simulink model "TeamA_PAsqualo"  (R2020a)
settings: Solver=VariableStepAuto  StartTime=0.0  StopTime=stop_time  FixedStep=0.05  RelTol=1e-3
InitFcn:
  | main_init
values from neighbouring files (symbols this model uses):
  a1 = rho * D^4 * alpha1    (= 0.000388302366464)    [main_init.m]
  a2 = -rho * D^3 * alpha2 * (1 - omega)    (= 0.0037030698432)    [main_init.m]
  ag = [Ax Ay Az]'    [init_modello.m]
  alpha1 = 0.0113    [main_init.m]
  alpha2 = -0.0091    [main_init.m]
  areaOfInterestCorner = [42.317744;10.915136; 0]    [init_controllo.m]    (also in missionA.m = [42.317744)
  bg = [Bx By Bz]'    [init_modello.m]
  cd_pitch = 0.7    [init_modello.m]
  cd_roll = 0.04    [init_modello.m]
  cd_x = 0.4    [init_modello.m]
  cd_y = 1    [init_modello.m]
  cd_yaw = 0.7    [init_modello.m]
  cd_z = 1    [init_modello.m]
  cg = [Cx Cy Cz]'    [init_modello.m]
  D = 0.076    [main_init.m]
  dead_zone_limit = 31.5    [main_init.m]
  dg = [Dx Dy Dz]'    [init_modello.m]
  eg = [Ex Ey Ez]'    [init_modello.m]
  fg = [Fx Fy Fz]'    [init_modello.m]
  g = 9.81    [init_modello.m]
  galleggiamento = 7.6786    [init_controllo.m]
  gg = [Gx Gy Gz]'    [init_modello.m]
  H0 = 0    [init_modello.m]
  init_position = [pointP(1),pointP(2),0.15,0,0,deg2rad(alpha)]'    [init_modello.m]
  init_velocity = [0 0 0 0 0 0]'    [init_modello.m]
  initial_state_cov = blkdiag(diag(cov_gps(1,1:2)), cov_depth*eye(n_state_filter-2))    [init_navigazione.m]
  Ixx = 0.93304097392    [init_modello.m]
  Ixy = 0    [init_modello.m]
  Ixz = 0    [init_modello.m]
  Iyy = 25.58745481378    (= 25.5874548138)    [init_modello.m]
  Iyz = 0    [init_modello.m]
  Izz = 25.58745481378    (= 25.5874548138)    [init_modello.m]
  K_i_heave_div = 20    [init_controllo.m]
  K_i_heave_pos = 1    [init_controllo.m]
  K_i_heave_surf = 20    [init_controllo.m]
  K_i_heave_trans = 5    [init_controllo.m]
  K_i_heave_turn = 5    [init_controllo.m]
  K_i_pitch_div = 0    [init_controllo.m]
  K_i_pitch_pos = 0    [init_controllo.m]
  K_i_pitch_surf = 0    [init_controllo.m]
  K_i_pitch_trans = 0    [init_controllo.m]
  K_i_pitch_turn = 0    [init_controllo.m]
  K_i_roll_div = 0    [init_controllo.m]
  K_i_roll_pos = 0    [init_controllo.m]
  K_i_roll_surf = 1    [init_controllo.m]
  K_i_roll_trans = 0    [init_controllo.m]
  K_i_roll_turn = 0    [init_controllo.m]
  K_i_surge_div = 3    [init_controllo.m]
  K_i_surge_pos = 5    [init_controllo.m]
  K_i_surge_surf = 3    [init_controllo.m]
  K_i_surge_trans = 2.5    [init_controllo.m]
  K_i_surge_turn = 10    [init_controllo.m]
  K_i_sway_div = 6    [init_controllo.m]
  K_i_sway_pos = 5    [init_controllo.m]
  K_i_sway_surf = 3    [init_controllo.m]
  K_i_sway_trans = 6    [init_controllo.m]
  K_i_sway_turn = 50    [init_controllo.m]
  K_i_yaw_div = 0    [init_controllo.m]
  K_i_yaw_pos = 1    [init_controllo.m]
  K_i_yaw_surf = 0    [init_controllo.m]
  K_i_yaw_trans = 20    [init_controllo.m]
  K_p_heave_div = 200    [init_controllo.m]
  K_p_heave_pos = 350    [init_controllo.m]
  K_p_heave_surf = 200    [init_controllo.m]
  K_p_heave_trans = 200    [init_controllo.m]
  K_p_heave_turn = 200    [init_controllo.m]
  K_p_phi_div = 0.15    [init_controllo.m]
  K_p_phi_pos = 0.1    [init_controllo.m]
  K_p_phi_surf = 0.15    [init_controllo.m]
  K_p_phi_trans = 0.1    [init_controllo.m]
  K_p_phi_turn = 0.1    [init_controllo.m]
  K_p_pitch_div = 50    [init_controllo.m]
  K_p_pitch_pos = 25    [init_controllo.m]
  K_p_pitch_surf = 50    [init_controllo.m]
  K_p_pitch_trans = 25    [init_controllo.m]
  K_p_pitch_turn = 25    [init_controllo.m]
  K_p_psi_div = 0.3    [init_controllo.m]
  K_p_psi_pos = 0.25    [init_controllo.m]
  K_p_psi_surf = 0.3    [init_controllo.m]
  K_p_psi_trans = 0.2    [init_controllo.m]
  K_p_roll_div = 10    [init_controllo.m]
  K_p_roll_pos = 4    [init_controllo.m]
  K_p_roll_surf = 10    [init_controllo.m]
  K_p_roll_trans = 4    [init_controllo.m]
  K_p_roll_turn = 4    [init_controllo.m]
  K_p_surge_div = 80    [init_controllo.m]
  K_p_surge_pos = 34.5    [init_controllo.m]
  K_p_surge_surf = 80    [init_controllo.m]
  K_p_surge_trans = 40    [init_controllo.m]
  K_p_surge_turn = 150    [init_controllo.m]
  K_p_sway_div = 100    [init_controllo.m]
  K_p_sway_pos = 90    [init_controllo.m]
  K_p_sway_surf = 80    [init_controllo.m]
  K_p_sway_trans = 90    [init_controllo.m]
  K_p_sway_turn = 200    [init_controllo.m]
  K_p_th_div = 0.3    [init_controllo.m]
  K_p_th_pos = 0.1    [init_controllo.m]
  K_p_th_surf = 0.3    [init_controllo.m]
  K_p_th_trans = 0.1    [init_controllo.m]
  K_p_th_turn = 0.1    [init_controllo.m]
  K_p_x_div = 0.12    [init_controllo.m]
  K_p_x_pos = 0.12    [init_controllo.m]
  K_p_x_surf = 0.12    [init_controllo.m]
  K_p_y_div = 0.6    [init_controllo.m]
  K_p_y_pos = 0.34    [init_controllo.m]
  K_p_y_surf = 0.1    [init_controllo.m]
  K_p_y_trans = 0.3    [init_controllo.m]
  K_p_y_turn = 0.3    [init_controllo.m]
  K_p_yaw_div = 70    [init_controllo.m]
  K_p_yaw_pos = 20    [init_controllo.m]
  K_p_yaw_surf = 70    [init_controllo.m]
  K_p_yaw_trans = 160    [init_controllo.m]
  K_p_z_div = 0.35    [init_controllo.m]
  K_p_z_pos = 0.2    [init_controllo.m]
  K_p_z_surf = 0.35    [init_controllo.m]
  K_p_z_trans = 0.7    [init_controllo.m]
  K_p_z_turn = 0.7    [init_controllo.m]
  Kadd = 0    [init_modello.m]
  m = 106    [init_modello.m]
  Madd = -((((1/5)*(b^2-a^2)^2))*(alpha_0-beta_0))/((((2*(b^2-a^2)^2))+(b^2-a^2)^2)*(alpha_0-beta_0)*m)    [init_modello.m]
  ... (+59 more)
undefined symbols (not defined in the file or in its folder): DiscIntNeverNeededParam, initial_state
libraries: simulink x2, vrlib x1
(part 5 of 5)

== matlab function TeamA_PAsqualo/controller/positioning controller/sway_controller/Sway PID controller/compute_position_errors ==
  data: enable input; err_pos output; ref input; est_state input; areaOfInterestCorner parameter
function err_pos = fcn(enable, ref, est_state,areaOfInterestCorner)
references_NED = zeros(3,1);
est_state_NED  = zeros(3,1);
phi = est_state(4);
th  = est_state(5);
psi = est_state(6);
coder.extrinsic('evalin','wgs84Ellipsoid','geodetic2ned');   
orig = [areaOfInterestCorner(1)   areaOfInterestCorner(2)   areaOfInterestCorner(3)]'; %origine terna NED
wgs84 = wgs84Ellipsoid;
if enable == 1
    % Cambiamento di riferimento da WGS84 a NED frame
   [x_ref, y_ref, z_ref] = geodetic2ned(ref(1),ref(2),ref(3),orig(1),orig(2),orig(3),wgs84);
   references_NED = [x_ref, y_ref, z_ref]';
   [x_est, y_est, z_est] = geodetic2ned(est_state(1),est_state(2),est_state(3),orig(1),orig(2),orig(3),wgs84);
   est_state_NED  =  [x_est, y_est, est_state(3)]';
   % Calcolo errore posizione da NED a BODY frame
   err_NED  = references_NED - est_state_NED;
   %
   R_z_psi = [cos(psi)    sin(psi)     0;
              -sin(psi)   cos(psi)     0;
                 0           0         1];
          
   R_y_th =  [cos(th)        0      -sin(th);
                 0           1         0;
              sin(th)        0       cos(th)];
       
   R_x_phi = [   1           0             0;
                 0         cos(phi)    sin(phi);
                 0        -sin(phi)    cos(phi)];
          
   R_NB = ((R_z_psi')*(R_y_th')*(R_x_phi'))'; % matrice rotazione NED->BODY
   err_pos_BODY = R_NB * err_NED;
   err_pos = err_pos_BODY(2);
else 
   err_pos = 0;
end
end

== matlab function TeamA_PAsqualo/controller/positioning controller/sway_controller/Sway PID controller/compute_velocity_error ==
  data: enable input; err_vel output; v_des input; est_meas input
function err_vel = fcn(enable,v_des,est_meas)
if enable == 1
   err_vel =  v_des - est_meas(8);

else 
    err_vel = 0;
end
end

== matlab function TeamA_PAsqualo/controller/positioning controller/yaw_controller/Yaw PID controller/compute_orientation_errors ==
  data: enable input; err_orient output; ref input; est_state input
function err_orient = fcn(enable, ref, est_state)
coder.extrinsic('wrapToPi');
err_orient = 0;
phi = est_state(4);
th  = est_state(5);
%
J_inv = [1       0          -sin(th); 
         0   cos(phi)  cos(th)*sin(phi);
         0  -sin(phi)  cos(th)*cos(phi)];
if enable == 1
   err_orient_1 = wrapToPi(J_inv*([ref(4);ref(5);ref(6)] -...
                           [est_state(4);est_state(5);est_state(6)]));
else 
   err_orient_1 = zeros(3,1);
end
err_orient = err_orient_1(3);
end

== matlab function TeamA_PAsqualo/controller/positioning controller/yaw_controller/Yaw PID controller/compute_velocity_error ==
  data: enable input; err_vel output; v_des input; est_meas input
function err_vel = fcn(enable,v_des,est_meas)
if enable == 1
   err_vel =  v_des - est_meas(12);
else
    err_vel = 0;
end
end

== matlab function TeamA_PAsqualo/controller/surfacing controller/heave_controller/Heave PID controller/compute_position_errors ==
  data: enable input; err_pos output; ref input; est_state input; w_des output; areaOfInterestCorner parameter
function [err_pos, w_des] = fcn(enable, ref, est_state,areaOfInterestCorner)
references_NED = zeros(3,1);
est_state_NED  = zeros(3,1);
phi = est_state(4);
th  = est_state(5);
psi = est_state(6);
coder.extrinsic('evalin','wgs84Ellipsoid','geodetic2ned');
orig = [areaOfInterestCorner(1)   areaOfInterestCorner(2)   areaOfInterestCorner(3)]'; %origine terna NED
wgs84 = wgs84Ellipsoid;
err_pos = 0;
w_des = 0;
if enable == 1
    % Cambiamento di riferimento da WGS84 a NED frame
   [x_ref, y_ref, z_ref] = geodetic2ned(ref(1),ref(2),ref(3),orig(1),orig(2),orig(3),wgs84);
   references_NED = [x_ref, y_ref, z_ref]';
   [x_est, y_est, z_est] = geodetic2ned(est_state(1),est_state(2),est_state(3),orig(1),orig(2),orig(3),wgs84);
   est_state_NED  =  [x_est, y_est, z_est]';
   est_state_NED = [est_state_NED(1);est_state_NED(2);est_state(3)];
   % Calcolo errore posizione da NED a BODY frame
   err_NED  = references_NED - est_state_NED;
   R_z_psi = [cos(psi)    sin(psi)     0;
              -sin(psi)   cos(psi)     0;
                 0           0         1];
          
   R_y_th =  [cos(th)        0      -sin(th);
                 0           1         0;
              sin(th)        0       cos(th)];
       
   R_x_phi = [   1           0             0;
                 0         cos(phi)    sin(phi);
                 0        -sin(phi)    cos(phi)];
          
   R_NB = ((R_z_psi')*(R_y_th')*(R_x_phi'))';
   err_pos_BODY = R_NB * err_NED;
   offset = -0.5;  % metri di distanza dal punto desiderato
   if err_pos_BODY(3) < offset
       err_pos = 0;
       w_des   = ref(9);
   end
   if err_pos_BODY(3) > offset
       err_pos = err_pos_BODY(3);
       w_des   = 0;
   end
else
   err_pos = 0;
   w_des   = 0;
end
end

== matlab function TeamA_PAsqualo/controller/surfacing controller/pitch_controller/Pitch PID controller/compute_orientation_errors ==
  data: enable input; err_orient output; ref input; est_state input
function err_orient = fcn(enable, ref, est_state)
coder.extrinsic('wrapToPi');
err_orient = 0;
phi = est_state(4);
th  = est_state(5);
%
J_inv = [1       0          -sin(th); 
         0   cos(phi)  cos(th)*sin(phi);
         0  -sin(phi)  cos(th)*cos(phi)];
if enable == 1
   err_orient_1 = wrapToPi(J_inv*([ref(4);ref(5);ref(6)] -...
                           [est_state(4);est_state(5);est_state(6)]));
else 
   err_orient_1 = zeros(3,1);
end
err_orient = err_orient_1(2);
end

== matlab function TeamA_PAsqualo/controller/surfacing controller/pitch_controller/Pitch PID controller/compute_velocity_error ==
  data: enable input; err_vel output; v_des input; est_meas input
function err_vel = fcn(enable,v_des,est_meas)
if enable == 1
   err_vel =  v_des - est_meas(11);
else
    err_vel = 0;
end
end

== matlab function TeamA_PAsqualo/controller/surfacing controller/heave_controller/Heave PID controller/compute_velocity_error ==
  data: enable input; err_vel output; v_des input; est_meas input
function err_vel = fcn(enable,v_des,est_meas)
if enable == 1
   err_vel =  v_des - est_meas(9);
else
    err_vel = 0;
end
end

== matlab function TeamA_PAsqualo/controller/surfacing controller/roll_controller/Roll PID controller/compute_orientation_errors ==
  data: enable input; err_orient output; ref input; est_state input
function err_orient = fcn(enable, ref, est_state)
coder.extrinsic('wrapToPi');
err_orient = 0;
phi = est_state(4);
th  = est_state(5);
%
J_inv = [1       0          -sin(th); 
         0   cos(phi)  cos(th)*sin(phi);
         0  -sin(phi)  cos(th)*cos(phi)];
if enable == 1
   err_orient_1 = wrapToPi(J_inv*([ref(4);ref(5);ref(6)] -...
                           [est_state(4);est_state(5);est_state(6)]));
else 
   err_orient_1 = zeros(3,1);
end
err_orient = err_orient_1(1);
end

== matlab function TeamA_PAsqualo/controller/surfacing controller/roll_controller/Roll PID controller/compute_velocity_error ==
  data: enable input; err_vel output; v_des input; est_meas input
function err_vel = fcn(enable,v_des,est_meas)
if enable == 1
   err_vel =  v_des - est_meas(10);
else
    err_vel = 0;
end
end

== matlab function TeamA_PAsqualo/controller/surfacing controller/surge_controller/Surge PID controller/compute_position_errors ==
  data: enable input; err_pos output; ref input; est_state input; areaOfInterestCorner parameter
function err_pos = fcn(enable, ref, est_state,areaOfInterestCorner)
references_NED = zeros(3,1);
est_state_NED  = zeros(3,1);
phi = est_state(4);
th  = est_state(5);
psi = est_state(6);
coder.extrinsic('evalin','wgs84Ellipsoid','geodetic2ned');
orig = [areaOfInterestCorner(1)   areaOfInterestCorner(2)   areaOfInterestCorner(3)]'; %origine terna NED
wgs84 = wgs84Ellipsoid;
if enable == 1
    % Cambiamento di riferimento da WGS84 a NED frame
   [x_ref, y_ref, z_ref] = geodetic2ned(ref(1),ref(2),ref(3),orig(1),orig(2),orig(3),wgs84);
   references_NED = [x_ref, y_ref, z_ref]';
   [x_est, y_est, z_est] = geodetic2ned(est_state(1),est_state(2),est_state(3),orig(1),orig(2),orig(3),wgs84);
   est_state_NED  =  [x_est, y_est, est_state(3)]';
   % Calcolo errore posizione da NED a BODY frame
   err_NED  = references_NED - est_state_NED;
   R_z_psi = [cos(psi)    sin(psi)     0;
              -sin(psi)   cos(psi)     0;
                 0           0         1];
          
   R_y_th =  [cos(th)        0      -sin(th);
                 0           1         0;
              sin(th)        0       cos(th)];
       
   R_x_phi = [   1           0             0;
                 0         cos(phi)    sin(phi);
                 0        -sin(phi)    cos(phi)];
          
   R_NB = ((R_z_psi')*(R_y_th')*(R_x_phi'))';
   err_pos_BODY = R_NB * err_NED;
   err_pos = err_pos_BODY(1);
else
   err_pos = 0;
end
end

== matlab function TeamA_PAsqualo/controller/surfacing controller/surge_controller/Surge PID controller/compute_velocity_error ==
  data: enable input; err_vel output; v_des input; est_meas input
function err_vel = fcn(enable,v_des,est_meas)
if enable == 1
   err_vel =  v_des - est_meas(7);
else
    err_vel = 0;
end
end

== matlab function TeamA_PAsqualo/controller/surfacing controller/sway_controller/Sway PID controller/compute_position_errors ==
  data: enable input; err_pos output; ref input; est_state input; areaOfInterestCorner parameter
function err_pos = fcn(enable, ref, est_state,areaOfInterestCorner)
references_NED = zeros(3,1);
est_state_NED  = zeros(3,1);
phi = est_state(4);
th  = est_state(5);
psi = est_state(6);
coder.extrinsic('evalin','wgs84Ellipsoid','geodetic2ned');
orig = [areaOfInterestCorner(1)   areaOfInterestCorner(2)   areaOfInterestCorner(3)]'; %origine terna NED
wgs84 = wgs84Ellipsoid;
if enable == 1
    % Cambiamento di riferimento da WGS84 a NED frame
   [x_ref, y_ref, z_ref] = geodetic2ned(ref(1),ref(2),ref(3),orig(1),orig(2),orig(3),wgs84);
   references_NED = [x_ref, y_ref, z_ref]';
   [x_est, y_est, z_est] = geodetic2ned(est_state(1),est_state(2),est_state(3),orig(1),orig(2),orig(3),wgs84);
   est_state_NED  =  [x_est, y_est,est_state(3)]';
   % Calcolo errore posizione da NED a BODY frame
   err_NED  = references_NED - est_state_NED;
   R_z_psi = [cos(psi)    sin(psi)     0;
              -sin(psi)   cos(psi)     0;
                 0           0         1];
          
   R_y_th =  [cos(th)        0      -sin(th);
                 0           1         0;
              sin(th)        0       cos(th)];
       
   R_x_phi = [   1           0             0;
                 0         cos(phi)    sin(phi);
                 0        -sin(phi)    cos(phi)];
          
   R_NB = ((R_z_psi')*(R_y_th')*(R_x_phi'))';
   err_pos_BODY = R_NB * err_NED;
   err_pos = err_pos_BODY(2);
else
   err_pos = 0;
end
end

== matlab function TeamA_PAsqualo/controller/surfacing controller/sway_controller/Sway PID controller/compute_velocity_error ==
  data: enable input; err_vel output; v_des input; est_meas input
function err_vel = fcn(enable,v_des,est_meas)
if enable == 1
   err_vel =  v_des - est_meas(8);
else
    err_vel = 0;
end
end

== matlab function TeamA_PAsqualo/controller/surfacing controller/yaw_controller/Yaw PID controller/compute_orientation_errors ==
  data: enable input; err_orient output; ref input; est_state input
function err_orient = fcn(enable, ref, est_state)
coder.extrinsic('wrapToPi');
err_orient = 0;
phi = est_state(4);
th  = est_state(5);
%
J_inv = [1       0          -sin(th); 
         0   cos(phi)  cos(th)*sin(phi);
         0  -sin(phi)  cos(th)*cos(phi)];
if enable == 1
   err_orient_1 = wrapToPi(J_inv*([ref(4);ref(5);ref(6)] -...
                           [est_state(4);est_state(5);est_state(6)]));
else 
   err_orient_1 = zeros(3,1);
end
err_orient = err_orient_1(3);
end

== matlab function TeamA_PAsqualo/controller/surfacing controller/yaw_controller/Yaw PID controller/compute_velocity_error ==
  data: enable input; err_vel output; v_des input; est_meas input
function err_vel = fcn(enable,v_des,est_meas)
if enable == 1
   err_vel =  v_des - est_meas(12);
else
    err_vel = 0;
end
end

== matlab function TeamA_PAsqualo/controller/transect controller/heave_controller/Heave PID controller/compute_position_errors ==
  data: enable input; err_pos output; ref input; est_state input; areaOfInterestCorner parameter
function err_pos = fcn(enable, ref, est_state,areaOfInterestCorner)
references_NED = zeros(3,1);
est_state_NED  = zeros(3,1);
phi = est_state(4);
th  = est_state(5);
psi = est_state(6);
coder.extrinsic('evalin','wgs84Ellipsoid','geodetic2ned');
orig = [areaOfInterestCorner(1)   areaOfInterestCorner(2)   areaOfInterestCorner(3)]'; %origine terna NED
wgs84 = wgs84Ellipsoid;
if enable == 1
    % Cambiamento di riferimento da WGS84 a NED frame
   [x_ref, y_ref, z_ref] = geodetic2ned(ref(1),ref(2),ref(3),orig(1),orig(2),orig(3),wgs84);
   references_NED = [x_ref, y_ref, z_ref]';
   [x_est, y_est, z_est] = geodetic2ned(est_state(1),est_state(2),est_state(3),orig(1),orig(2),orig(3),wgs84);
   est_state_NED  =  [x_est, y_est, z_est]';
   est_state_NED = [est_state_NED(1);est_state_NED(2);est_state(3)];
   % Calcolo errore posizione da NED a BODY frame
   err_NED  = references_NED - est_state_NED;
   R_z_psi = [cos(psi)    sin(psi)     0;
              -sin(psi)   cos(psi)     0;
                 0           0         1];
          
   R_y_th =  [cos(th)        0      -sin(th);
                 0           1         0;
              sin(th)        0       cos(th)];
       
   R_x_phi = [   1           0             0;
                 0         cos(phi)    sin(phi);
                 0        -sin(phi)    cos(phi)];
          
   R_NB = ((R_z_psi')*(R_y_th')*(R_x_phi'))';
   err_pos_BODY = R_NB * err_NED;
   err_pos = err_pos_BODY(3);
else
   err_pos = 0;
end
end

== matlab function TeamA_PAsqualo/controller/transect controller/heave_controller/Heave PID controller/compute_velocity_error ==
  data: enable input; err_vel output; v_des input; est_meas input
function err_vel = fcn(enable,v_des,est_meas)
if enable == 1
   err_vel =  v_des - est_meas(9);
else
    err_vel = 0;
end
end

== matlab function TeamA_PAsqualo/controller/transect controller/pitch_controller/Pitch PID controller/compute_orientation_errors ==
  data: enable input; err_orient output; ref input; est_state input
function err_orient = fcn(enable, ref, est_state)
coder.extrinsic('wrapToPi');
err_orient = 0;
phi = est_state(4);
th  = est_state(5);
%
J_inv = [1       0          -sin(th); 
         0   cos(phi)  cos(th)*sin(phi);
         0  -sin(phi)  cos(th)*cos(phi)];
if enable == 1
   err_orient_1 = wrapToPi(J_inv*([ref(4);ref(5);ref(6)] -...
                           [est_state(4);est_state(5);est_state(6)]));
else 
   err_orient_1 = zeros(3,1);
end
err_orient = err_orient_1(2);
end

== matlab function TeamA_PAsqualo/controller/transect controller/pitch_controller/Pitch PID controller/compute_velocity_error ==
  data: enable input; err_vel output; v_des input; est_meas input
function err_vel = fcn(enable,v_des,est_meas)
if enable == 1
   err_vel =  v_des - est_meas(11);
else
    err_vel = 0;
end
end

== matlab function TeamA_PAsqualo/controller/transect controller/roll_controller/Roll PID controller/compute_orientation_errors ==
  data: enable input; err_orient output; ref input; est_state input
function err_orient = fcn(enable, ref, est_state)
coder.extrinsic('wrapToPi');
err_orient = 0;
phi = est_state(4);
th  = est_state(5);
%
J_inv = [1       0          -sin(th); 
         0   cos(phi)  cos(th)*sin(phi);
         0  -sin(phi)  cos(th)*cos(phi)];
if enable == 1
   err_orient_1 = wrapToPi(J_inv*([ref(4);ref(5);ref(6)] -...
                           [est_state(4);est_state(5);est_state(6)]));
else 
   err_orient_1 = zeros(3,1);
end
err_orient = err_orient_1(1);
end

== matlab function TeamA_PAsqualo/controller/transect controller/roll_controller/Roll PID controller/compute_velocity_error ==
  data: enable input; err_vel output; v_des input; est_meas input
function err_vel = fcn(enable,v_des,est_meas)
if enable == 1
   err_vel =  v_des - est_meas(10);
else
    err_vel = 0;
end
end

== matlab function TeamA_PAsqualo/controller/transect controller/surge_controller/Surge PID controller/ compute_velocity_error ==
  data: enable input; ref input; est_meas input; err_vel output
function err_vel = fcn(enable, ref, est_meas)
if  enable == 1
    err_vel = ref(7) - est_meas(7);
else
    err_vel = 0;
end
end

== matlab function TeamA_PAsqualo/controller/transect controller/sway_controller/Sway PID controller/compute_position_errors ==
  data: enable input; err_pos output; ref input; est_state input; areaOfInterestCorner parameter
function err_pos = fcn(enable, ref, est_state,areaOfInterestCorner)
coder.extrinsic('wrapToPi');
coder.extrinsic('evalin','wgs84Ellipsoid','geodetic2ned');
references_NED = zeros(3,1);
est_state_NED  = zeros(3,1);
phi = est_state(4);
th  = est_state(5);
psi = est_state(6);
psi = wrapToPi(psi);
orig = [areaOfInterestCorner(1)   areaOfInterestCorner(2)   areaOfInterestCorner(3)]'; %origine terna NED
wgs84 = wgs84Ellipsoid;
if enable == 1
    % Cambiamento di riferimento da WGS84 a NED frame
   [x_ref, y_ref, z_ref] = geodetic2ned(ref(1),ref(2),ref(3),orig(1),orig(2),orig(3),wgs84);
   references_NED = [x_ref, y_ref, z_ref]';
   [x_est, y_est, z_est] = geodetic2ned(est_state(1),est_state(2),est_state(3),orig(1),orig(2),orig(3),wgs84);
   est_state_NED  =  [x_est, y_est, est_state(3)]';
   % Calcolo errore posizione da NED a BODY frame
   err_NED  = references_NED - est_state_NED;
   R_z_psi = [cos(psi)    sin(psi)     0;
              -sin(psi)   cos(psi)     0;
                 0           0         1];
          
   R_y_th =  [cos(th)        0      -sin(th);
                 0           1         0;
              sin(th)        0       cos(th)];
       
   R_x_phi = [   1           0             0;
                 0         cos(phi)    sin(phi);
                 0        -sin(phi)    cos(phi)];
          
   R_NB = ((R_z_psi')*(R_y_th')*(R_x_phi'))';
   err_pos_BODY = R_NB * err_NED;
   err_pos = err_pos_BODY(2);
else
   err_pos = 0;
end
end

== matlab function TeamA_PAsqualo/controller/transect controller/sway_controller/Sway PID controller/compute_velocity_error ==
  data: enable input; err_vel output; v_des input; est_meas input
function err_vel = fcn(enable,v_des,est_meas)
if enable == 1
   err_vel =  v_des - est_meas(8);
else
    err_vel = 0;
end
end

== matlab function TeamA_PAsqualo/controller/transect controller/yaw_controller/Yaw PID controller/compute_orientation_errors ==
  data: enable input; err_orient output; ref input; est_state input
function err_orient = fcn(enable, ref, est_state)
coder.extrinsic('wrapToPi');
err_orient = 0;
phi = est_state(4);
th  = est_state(5);
%
J_inv = [1       0          -sin(th); 
         0   cos(phi)  cos(th)*sin(phi);
         0  -sin(phi)  cos(th)*cos(phi)];
if enable == 1
   err_orient_1 = wrapToPi(J_inv*([ref(4);ref(5);ref(6)] -...
                           [est_state(4);est_state(5);est_state(6)]));
else 
   err_orient_1 = zeros(3,1);
end
err_orient = err_orient_1(3);
end

== matlab function TeamA_PAsqualo/controller/transect controller/yaw_controller/Yaw PID controller/compute_velocity_error ==
  data: enable input; err_vel output; v_des input; est_meas input
function err_vel = fcn(enable,v_des,est_meas)
if enable == 1
   err_vel =  v_des - est_meas(12);
else
    err_vel = 0;
end
end

== matlab function TeamA_PAsqualo/controller/turning controller/heave_controller/Heave PID controller/compute_position_errors ==
  data: enable input; err_pos output; ref input; est_state input; areaOfInterestCorner parameter
function err_pos = fcn(enable, ref, est_state,areaOfInterestCorner)
references_NED = zeros(3,1);
est_state_NED  = zeros(3,1);
phi = est_state(4);
th  = est_state(5);
psi = est_state(6);
coder.extrinsic('evalin','wgs84Ellipsoid','geodetic2ned');
orig = [areaOfInterestCorner(1)   areaOfInterestCorner(2)   areaOfInterestCorner(3)]'; %origine terna NED
wgs84 = wgs84Ellipsoid;
if enable == 1
   % Cambiamento di riferimento da WGS84 a NED frame
   [x_ref, y_ref, z_ref] = geodetic2ned(ref(1),ref(2),ref(3),orig(1),orig(2),orig(3),wgs84);
   references_NED = [x_ref, y_ref, z_ref]';
   [x_est, y_est, z_est] = geodetic2ned(est_state(1),est_state(2),est_state(3),orig(1),orig(2),orig(3),wgs84);
   est_state_NED  =  [x_est, y_est, z_est]';
   est_state_NED = [est_state_NED(1);est_state_NED(2);est_state(3)];
   % Calcolo errore posizione da NED a BODY frame
   err_NED  = references_NED - est_state_NED;
   R_z_psi = [cos(psi)    sin(psi)     0;
              -sin(psi)   cos(psi)     0;
                 0           0         1];
          
   R_y_th =  [cos(th)        0      -sin(th);
                 0           1         0;
              sin(th)        0       cos(th)];
       
   R_x_phi = [   1           0             0;
                 0         cos(phi)    sin(phi);
                 0        -sin(phi)    cos(phi)];
          
   R_NB = ((R_z_psi')*(R_y_th')*(R_x_phi'))';
   err_pos_BODY = R_NB * err_NED;
   err_pos = err_pos_BODY(3);
else
   err_pos = 0;
end
end

== matlab function TeamA_PAsqualo/controller/turning controller/heave_controller/Heave PID controller/compute_velocity_error ==
  data: enable input; err_vel output; v_des input; est_meas input
function err_vel = fcn(enable,v_des,est_meas)
if enable == 1
   err_vel =  v_des - est_meas(9);
else
    err_vel = 0;
end
end

== matlab function TeamA_PAsqualo/controller/turning controller/pitch_controller/Pitch PID controller/compute_orientation_errors ==
  data: enable input; err_orient output; ref input; est_state input
function err_orient = fcn(enable, ref, est_state)
coder.extrinsic('wrapToPi');
err_orient = 0;
phi = est_state(4);
th  = est_state(5);
%
J_inv = [1       0          -sin(th); 
         0   cos(phi)  cos(th)*sin(phi);
         0  -sin(phi)  cos(th)*cos(phi)];
if enable == 1
   err_orient_1 = wrapToPi(J_inv*([ref(4);ref(5);ref(6)] -...
                           [est_state(4);est_state(5);est_state(6)]));
else 
   err_orient_1 = zeros(3,1);
end
err_orient = err_orient_1(2);
end

== matlab function TeamA_PAsqualo/controller/turning controller/pitch_controller/Pitch PID controller/compute_velocity_error ==
  data: enable input; err_vel output; v_des input; est_meas input
function err_vel = fcn(enable,v_des,est_meas)
if enable == 1
   err_vel =  v_des - est_meas(11);
else
    err_vel = 0;
end
end

== matlab function TeamA_PAsqualo/controller/turning controller/roll_controller/Roll PID controller/compute_orientation_errors ==
  data: enable input; err_orient output; ref input; est_state input
function err_orient = fcn(enable, ref, est_state)
coder.extrinsic('wrapToPi');
err_orient = 0;
phi = est_state(4);
th  = est_state(5);
%
J_inv = [1       0          -sin(th); 
         0   cos(phi)  cos(th)*sin(phi);
         0  -sin(phi)  cos(th)*cos(phi)];
if enable == 1
   err_orient_1 = wrapToPi(J_inv*([ref(4);ref(5);ref(6)] -...
                           [est_state(4);est_state(5);est_state(6)]));
else 
   err_orient_1 = zeros(3,1);
end
err_orient = err_orient_1(1);
end

== matlab function TeamA_PAsqualo/controller/turning controller/roll_controller/Roll PID controller/compute_velocity_error ==
  data: enable input; err_vel output; v_des input; est_meas input
function err_vel = fcn(enable,v_des,est_meas)
if enable == 1
   err_vel =  v_des - est_meas(10);
else
    err_vel = 0;
end
end

== matlab function TeamA_PAsqualo/controller/turning controller/surge_controller/Surge PID controller/ compute_velocity_error ==
  data: enable input; ref input; est_meas input; err_vel output
function err_vel = fcn(enable, ref, est_meas)
if  enable == 1
    err_vel = ref(7) - est_meas(7);
else
    err_vel = 0;
end
end

== matlab function TeamA_PAsqualo/controller/turning controller/sway_controller/Sway PID controller/compute_position_errors ==
  data: enable input; err_pos output; ref input; est_state input; areaOfInterestCorner parameter
function err_pos = fcn(enable, ref, est_state,areaOfInterestCorner)
references_NED = zeros(3,1);
est_state_NED  = zeros(3,1);
phi = est_state(4);
th  = est_state(5);
psi = est_state(6);
coder.extrinsic('evalin','wgs84Ellipsoid','geodetic2ned'); 
orig = [areaOfInterestCorner(1)   areaOfInterestCorner(2)   areaOfInterestCorner(3)]'; %origine terna NED
wgs84 = wgs84Ellipsoid;
if enable == 1
    % Cambiamento di riferimento da WGS84 a NED frame
   [x_ref, y_ref, z_ref] = geodetic2ned(ref(1),ref(2),ref(3),orig(1),orig(2),orig(3),wgs84);
   references_NED = [x_ref, y_ref, z_ref]';
   [x_est, y_est, z_est] = geodetic2ned(est_state(1),est_state(2),est_state(3),orig(1),orig(2),orig(3),wgs84);
   est_state_NED  =  [x_est, y_est, est_state(3)]';
   % Calcolo errore posizione da NED a BODY frame, con componente east
   err_NED  = references_NED - est_state_NED;
   R_z_psi = [cos(psi)    sin(psi)     0;
              -sin(psi)   cos(psi)     0;
                 0           0         1];
          
   R_y_th =  [cos(th)        0      -sin(th);
                 0           1         0;
              sin(th)        0       cos(th)];
       
   R_x_phi = [   1           0             0;
                 0         cos(phi)    sin(phi);
                 0        -sin(phi)    cos(phi)];
          
   R_NB = ((R_z_psi')*(R_y_th')*(R_x_phi'))';
   err_pos_BODY = R_NB * err_NED;
   err_pos = err_pos_BODY(2);
else
   err_pos = 0;
end
end

== matlab function TeamA_PAsqualo/controller/turning controller/sway_controller/Sway PID controller/compute_velocity_error ==
  data: enable input; err_vel output; v_des input; est_meas input
function err_vel = fcn(enable,v_des,est_meas)
if enable == 1
   err_vel =  v_des - est_meas(8);
else
    err_vel = 0;
end
end

== matlab function TeamA_PAsqualo/controller/turning controller/yaw_controller/Yaw PID controller/compute_orientation_errors ==
  data: enable input; err_orient output; ref input; est_state input
function err_orient = fcn(enable, ref, est_state)
coder.extrinsic('wrapToPi');
err_orient = 0;
phi = est_state(4);
th  = est_state(5);
%
J_inv = [1       0          -sin(th); 
         0   cos(phi)  cos(th)*sin(phi);
         0  -sin(phi)  cos(th)*cos(phi)];
if enable == 1
   err_orient_1 = wrapToPi(J_inv*([ref(4);ref(5);ref(6)] -...
                           [est_state(4);est_state(5);est_state(6)]));
else 
   err_orient_1 = zeros(3,1);
end
err_orient = err_orient_1(3);
end

== matlab function TeamA_PAsqualo/Navigazione/MATLAB Function ==
  data: u input size=[3,1]; y output
function y = fcn(u)

if norm(u) > 1e5
	y = 0;
else
	y = 1;
end

end

== matlab function TeamA_PAsqualo/MATLAB Function1 ==
  data: pos_usbl output; USBL_Bearing_elevation input; USBL_Range input; pos_transp parameter
function pos_usbl = usblned(USBL_Bearing_elevation, USBL_Range, pos_transp)

pos_usbl = zeros(2,1);
posA2T = zeros(2,1);
posA2T(1) = cos(USBL_Bearing_elevation(1)) * cos(USBL_Bearing_elevation(2)) * USBL_Range;
posA2T(2) = sin(USBL_Bearing_elevation(1)) * cos(USBL_Bearing_elevation(2)) * USBL_Range;

pos_usbl(1) = pos_transp(1) - posA2T(1);
pos_usbl(2) = pos_transp(2) - posA2T(2);


end

== matlab function TeamA_PAsqualo/controller/turning controller/yaw_controller/Yaw PID controller/compute_velocity_error ==
  data: enable input; err_vel output; v_des input; est_meas input
function err_vel = fcn(enable,v_des,est_meas)
if enable == 1
   err_vel =  v_des - est_meas(12);
else
    err_vel = 0;
end
end

== matlab function TeamA_PAsqualo/geo2ned2 ==
  data: geo input; ned output size=[3 1]; ned_origin parameter
function ned = geo2ned(geo, ned_origin)
coder.extrinsic('evalin', 'wgs84Ellipsoid', 'geodetic2ned');

[x, y, ~] = geodetic2ned(geo(1), geo(2), -geo(3),ned_origin(1), ned_origin(2), ned_origin(3), wgs84Ellipsoid);

ned = zeros(3,1);
ned = [x;y;geo(3)];
end

== matlab function TeamA_PAsqualo/Sensors and Environment Models /Global Positioning System/MATLAB Function ==
  data: ned input; position output
function position = ned2wgs84(ned)

coder.extrinsic('evalin', 'ned2geodetic', 'wgs84Ellipsoid');
position = [0;0;0];
NED_origin = [0;0;0];
NED_origin = evalin('base', 'NED_origin');
[a b c] = ned2geodetic(ned(1), ned(2), ned(3), NED_origin(1), NED_origin(2),NED_origin(3), wgs84Ellipsoid);
position = [a; b; c];

end

== matlab function TeamA_PAsqualo/geo2ned3 ==
  data: geo input; ned output size=[3 1]; ned_origin parameter
function ned = geo2ned(geo, ned_origin)
coder.extrinsic('evalin', 'wgs84Ellipsoid', 'geodetic2ned');

[x, y, ~] = geodetic2ned(geo(1), geo(2), -geo(3),ned_origin(1), ned_origin(2), ned_origin(3), wgs84Ellipsoid);

ned = zeros(3,1);
ned = [x;y;geo(3)];
end

== matlab function TeamA_PAsqualo/controller/abort mission/abort mission ==
  data: enable input; abort output size=[6 1]; ref input; est_meas input
function abort = fcn(enable, ref, est_meas)
tau = zeros(6,1);
abort = zeros(6,1);
if enable == 1
    abort = tau;
else
    abort = tau;
end
end

== matlab function TeamA_PAsqualo/Vehicle Model/Thruster A/MATLAB Function ==
  data: n input; T output; V input; D parameter; omega parameter; a1 parameter; a2 parameter; alpha1 parameter; alpha2 parameter
function T = thrusterModel(n, V, D, omega, a1, a2, alpha1, alpha2)

Va = (1-omega) * V;     % Advancement velocity at the propeller
J0 = Va/(n*D);          % Advancement Coefficient

if J0 > -alpha1/alpha2  % Out of linearity domain (right side)
    T = 0;              % A null generated thrust is assumed
    
elseif J0 < 0           % Out of linearity domain (left side)
    T = a1*abs(n)*n;    % Bollard thrust is assumed

else                    % Within the linearity domain
    T = a1*abs(n)*n - a2*abs(n)*V;
end

== matlab function TeamA_PAsqualo/Vehicle Model/Thruster B/MATLAB Function ==
  data: n input; T output; V input; D parameter; omega parameter; a1 parameter; a2 parameter; alpha1 parameter; alpha2 parameter
function T = thrusterModel(n, V, D, omega, a1, a2, alpha1, alpha2)

Va = (1-omega) * V;     % Advancement velocity at the propeller
J0 = Va/(n*D);          % Advancement Coefficient

if J0 > -alpha1/alpha2  % Out of linearity domain (right side)
    T = 0;              % A null generated thrust is assumed
    
elseif J0 < 0           % Out of linearity domain (left side)
    T = a1*abs(n)*n;    % Bollard thrust is assumed

else                    % Within the linearity domain
    T = a1*abs(n)*n - a2*abs(n)*V;
end

== matlab function TeamA_PAsqualo/Vehicle Model/Thruster C/MATLAB Function ==
  data: n input; T output; V input; D parameter; omega parameter; a1 parameter; a2 parameter; alpha1 parameter; alpha2 parameter
function T = thrusterModel(n, V, D, omega, a1, a2, alpha1, alpha2)

Va = (1-omega) * V;     % Advancement velocity at the propeller
J0 = Va/(n*D);          % Advancement Coefficient

if J0 > -alpha1/alpha2  % Out of linearity domain (right side)
    T = 0;              % A null generated thrust is assumed
    
elseif J0 < 0           % Out of linearity domain (left side)
    T = a1*abs(n)*n;    % Bollard thrust is assumed

else                    % Within the linearity domain
    T = a1*abs(n)*n - a2*abs(n)*V;
end

== matlab function TeamA_PAsqualo/Vehicle Model/TAM ==
  data: Ta input; tau output double size=[6 1]; Tb input; Tc input; Td input; Te input; Tf input; Tg input; TAM parameter; eta input
function tau = fcn(Ta,Tb,Tc,Td,Te,Tf,Tg,TAM,eta)
thrust_vect = [Ta,Tb,Tc,Td,Te,Tf,Tg]';
if eta(3) >= 0
    tau = TAM*thrust_vect;
else
    tau = [0 0 0 0 0 0]';
end
end

== matlab function TeamA_PAsqualo/Vehicle Model/Thruster D/MATLAB Function ==
  data: n input; T output; V input; D parameter; omega parameter; a1 parameter; a2 parameter; alpha1 parameter; alpha2 parameter
function T = thrusterModel(n, V, D, omega, a1, a2, alpha1, alpha2)

Va = (1-omega) * V;     % Advancement velocity at the propeller
J0 = Va/(n*D);          % Advancement Coefficient

if J0 > -alpha1/alpha2  % Out of linearity domain (right side)
    T = 0;              % A null generated thrust is assumed
    
elseif J0 < 0           % Out of linearity domain (left side)
    T = a1*abs(n)*n;    % Bollard thrust is assumed

else                    % Within the linearity domain
    T = a1*abs(n)*n - a2*abs(n)*V;
end

== matlab function TeamA_PAsqualo/Vehicle Model/NED to LLDepth ==
  data: eta input double size=[6 1]; areaOfInterestCorner parameter; pos_true output double size=[3 1]; H0 parameter
function pos_true = fcn(eta,areaOfInterestCorner,H0)
coder.extrinsic('wgs84Ellipsoid');    % Reference spheroid
coder.extrinsic('ned2geodetic');
wgs84 = wgs84Ellipsoid('meter');
pos_true = zeros(3,1);
xNorth = eta(1);
yEast = eta(2);
zDown = eta(3);
LAT_AOIC = areaOfInterestCorner(1);
LON_AOIC = areaOfInterestCorner(2);
[Lat, Lon] = ned2geodetic(xNorth, yEast, zDown, LAT_AOIC, LON_AOIC, H0, wgs84,'degrees');
depth = zDown;
pos_true = [Lat, Lon, depth]';
end

== matlab function TeamA_PAsqualo/Vehicle Model/Coriolis computation ==
  data: nir input; C_effect output double size=[6 1]; m parameter; Ixx parameter; Iyy parameter; Izz parameter; Ixy parameter; Ixz parameter; Iyz parameter; Zadd parameter; Yadd parameter; Xadd parameter; Madd parameter; Nadd parameter; Kadd parameter
function C_effect = fcn(nir, m, Ixx, Iyy, Izz, Ixy, Ixz, Iyz, Zadd, Yadd, Xadd, Madd, Nadd, Kadd)
u = nir(1);
v = nir(2);
w = nir(3);
p = nir(4);
q = nir(5);
r = nir(6);

C11RB = zeros(3);
C12RB = m*[0 w -v;-w 0 u;v -u 0];
C21RB = -C12RB';
C22RB = [0 (-Iyz*q-Ixz*p+Izz*r) (Iyz*r+Ixy*p-Iyy*q);(Iyz*q+Ixz*p-Izz*r) 0 (-Ixz*r-Ixy*q+Ixx*p);-(Iyz*r+Ixy*p-Iyy*q) (Ixz*r+Ixy*q-Ixx*p) 0];
Crb = [C11RB C12RB;C21RB C22RB];

CA11 = zeros(3);
CA12 = [0 -Zadd*w Yadd*v;Zadd*w 0 -Xadd*u;-Yadd*v Xadd*u 0];
CA21 = -CA12';
CA22 = [0 -Nadd*r Madd*q;Nadd*r 0 -Kadd*p;-Madd*q Kadd*p 0];
Ca = [CA11 CA12;CA21 CA22];

C = Crb+Ca;
C_effect = C*nir;
end

== matlab function TeamA_PAsqualo/Vehicle Model/Damping computation ==
  data: nir input; D_effect output double size=[6 1]; cd_x parameter; cd_y parameter; cd_z parameter; cd_roll parameter; cd_pitch parameter; cd_yaw parameter; S_x parameter; S_y parameter; S_z parameter; S_roll parameter; S_pitch parameter; r_mz parameter; r_my parameter; r_mx parameter; S_yaw parameter; rho parameter
function D_effect = fcn(nir, cd_x, cd_y, cd_z, cd_roll, cd_pitch, cd_yaw, S_x, S_y, S_z, S_roll, S_pitch, r_mz, r_my, r_mx, S_yaw, rho)
%Calcolo matrice di Damping

vx = abs(nir(1));
vy = abs(nir(2));
vz = abs(nir(3));
wr = abs(nir(4));
wp = abs(nir(5));
wy = abs(nir(6));

D_x = -(1/2)*rho*cd_x*S_x*vx; %kg/m^3 * m^2 * m/s = kg/s (*m/s = N)
D_y = -(1/2)*rho*cd_y*S_y*vy;
D_z = -(1/2)*rho*cd_z*S_z*vz;

D_r = -(1/2)*rho*cd_roll*S_roll*((r_mx)^3)*wr; %kg/m^3 * m^2 * m^3 * 1/s = kg*m^2/s (*1/s = Nm)
D_p = -(1/2)*rho*cd_pitch*S_pitch*((r_my)^3)*wp;
D_yaw = -(1/2)*rho*cd_yaw*S_yaw*((r_mz)^3)*wy;

D = -blkdiag(D_x,D_y,D_z,D_r,D_p,D_yaw);

D_effect = D*nir;
end

== matlab function TeamA_PAsqualo/Vehicle Model/Gravity computation ==
  data: g_effect output double size=[6 1]; J1 input double size=[3 3]; Rb parameter; Rg parameter; W parameter; eta input; V parameter; rho parameter; g parameter
function g_effect = fcn(J1, Rb, Rg, W, eta,V, rho, g)
B = V*rho*g*[0 0 -1]'; %Forza galleggiamento in terna NED
J1_inv = inv(J1);
Fw = J1_inv*W; %Peso in terna Body
if eta(3) < -0.15
    Fb = [0,0,0]';
else
    if eta(3) <= 0.15
        B = ((eta(3)+0.15)/0.3)*B;
        Fb = J1_inv*B; %Galleggiamento in terna Body
    else
        Fb = J1_inv*B; %Galleggiamento in terna Body
    end
end
g_effect = -[Fw+Fb;cross(Rg,Fw)+cross(Rb,Fb)];
end

== matlab function TeamA_PAsqualo/Vehicle Model/Thruster E/MATLAB Function ==
  data: n input; T output; V input; D parameter; omega parameter; a1 parameter; a2 parameter; alpha1 parameter; alpha2 parameter
function T = thrusterModel(n, V, D, omega, a1, a2, alpha1, alpha2)

Va = (1-omega) * V;     % Advancement velocity at the propeller
J0 = Va/(n*D);          % Advancement Coefficient

if J0 > -alpha1/alpha2  % Out of linearity domain (right side)
    T = 0;              % A null generated thrust is assumed
    
elseif J0 < 0           % Out of linearity domain (left side)
    T = a1*abs(n)*n;    % Bollard thrust is assumed

else                    % Within the linearity domain
    T = a1*abs(n)*n - a2*abs(n)*V;
end

== matlab function TeamA_PAsqualo/Vehicle Model/Thruster F/MATLAB Function ==
  data: n input; T output; V input; D parameter; omega parameter; a1 parameter; a2 parameter; alpha1 parameter; alpha2 parameter
function T = thrusterModel(n, V, D, omega, a1, a2, alpha1, alpha2)

Va = (1-omega) * V;     % Advancement velocity at the propeller
J0 = Va/(n*D);          % Advancement Coefficient

if J0 > -alpha1/alpha2  % Out of linearity domain (right side)
    T = 0;              % A null generated thrust is assumed
    
elseif J0 < 0           % Out of linearity domain (left side)
    T = a1*abs(n)*n;    % Bollard thrust is assumed

else                    % Within the linearity domain
    T = a1*abs(n)*n - a2*abs(n)*V;
end

== matlab function TeamA_PAsqualo/Vehicle Model/MATLAB Function1 ==
  data: nir input double size=[6 1]; J1 input double size=[3 3]; ni_abs output double size=[6 1]; current_speed parameter double size=[3 1]
function ni_abs= fcn(nir,J1,current_speed)
J1_inv = inv(J1);
current_speed_Body = J1_inv*current_speed; %NED to Body computation
nir1 = [nir(1) nir(2) nir(3)]';
ni1_abs = nir1+current_speed_Body;
ni_abs = [ni1_abs(1) ni1_abs(2) ni1_abs(3) nir(4) nir(5) nir(6)]';
end

== matlab function TeamA_PAsqualo/Vehicle Model/J computation ==
  data: J output double size=[6 6]; eta input double size=[6 1]
function J  = fcn(eta)
phi = eta(4);
theta = eta(5);
psi = eta(6);
Rx = [1 0 0;0 cos(phi) sin(phi);0 -sin(phi) cos(phi)];
Ry = [cos(theta) 0 -sin(theta);0 1 0;sin(theta) 0 cos(theta)];
Rz = [cos(psi) sin(psi) 0;-sin(psi) cos(psi) 0; 0 0 1];
J1 = Rz'*Ry'*Rx';
J2_inv = [1 0 -sin(theta);0 cos(phi) (cos(theta)*sin(phi));0 -sin(phi) (cos(theta)*cos(phi))];
J2 = inv(J2_inv);
J = [J1 zeros(3);zeros(3) J2];
end

== matlab function TeamA_PAsqualo/Vehicle Model/MATLAB Function2 ==
  data: eta input double size=[6 1]; orient_true output
function orient_true = fcn(eta)
coder.extrinsic('wrapToPi');
orient_true = [0; 0; 0];
rr = eta(4);
r = wrapToPi(rr); %phi
pp = eta(5);
p = wrapToPi(pp); %theta
yy = eta(6);
y = wrapToPi(yy); %psi
orient_true = [r p y]';
end

== matlab function TeamA_PAsqualo/Vehicle Model/MATLAB Function3 ==
  data: ni_abs input double size=[6 1]; vel_true output double size=[3 1]
function vel_true = fcn(ni_abs)
vx = ni_abs(1);
vy = ni_abs(2);
vz = ni_abs(3);
vel_true = [vx,vy,vz]';
end

== matlab function TeamA_PAsqualo/Vehicle Model/MATLAB Function4 ==
  data: ni_abs input double size=[6 1]; w_true output double size=[3 1]
function w_true = fcn(ni_abs)
w_x = ni_abs(4);
w_y = ni_abs(5);
w_z = ni_abs(6);
w_true = [w_x,w_y,w_z]';
end

== matlab function TeamA_PAsqualo/Vehicle Model/Thruster G/MATLAB Function ==
  data: n input; T output; V input; D parameter; omega parameter; a1 parameter; a2 parameter; alpha1 parameter; alpha2 parameter
function T = thrusterModel(n, V, D, omega, a1, a2, alpha1, alpha2)

Va = (1-omega) * V;     % Advancement velocity at the propeller
J0 = Va/(n*D);          % Advancement Coefficient

if J0 > -alpha1/alpha2  % Out of linearity domain (right side)
    T = 0;              % A null generated thrust is assumed
    
elseif J0 < 0           % Out of linearity domain (left side)
    T = a1*abs(n)*n;    % Bollard thrust is assumed

else                    % Within the linearity domain
    T = a1*abs(n)*n - a2*abs(n)*V;
end

== matlab function TeamA_PAsqualo/Vehicle Model/Velocità_ai_thruster ==
  data: nir input double size=[6 1]; Va_rel output; Vb_rel output; Vc_rel output; Vd_rel output; Ve_rel output; Vf_rel output; Vg_rel output; orA parameter; orB parameter; orC parameter; orD parameter; orE parameter; orF parameter; orG parameter; ag parameter; bg parameter; cg parameter; dg parameter; eg parameter; fg parameter; gg parameter
function [Va_rel,Vb_rel,Vc_rel,Vd_rel,Ve_rel,Vf_rel,Vg_rel] = fcn(nir, orA, orB, orC, orD, orE, orF, orG, ag, bg, cg, dg, eg, fg, gg)
nir1 = [nir(1) nir(2) nir(3)]';
nir2 = [nir(4) nir(5) nir(6)]';
%Vettori orientazione thrusterX denominati orX  disponibili nel file init
%Vettori posizione thrusterX denominati xg disponibili nel file init
Va_rel = orA*(nir1 + cross(nir2,ag));
Vb_rel = orB*(nir1 + cross(nir2,bg));
Vc_rel = orC*(nir1 + cross(nir2,cg));
Vd_rel = orD*(nir1 + cross(nir2,dg));
Ve_rel = orE*(nir1 + cross(nir2,eg));
Vf_rel = orF*(nir1 + cross(nir2,fg));
Vg_rel = orG*(nir1 + cross(nir2,gg));
[Va_rel,Vb_rel,Vc_rel,Vd_rel,Ve_rel,Vf_rel,Vg_rel];
end
